simulink model "fibonachi_LFSR"  (R2024a)
settings: Solver=VariableStepAuto  StartTime=0.0  StopTime=1  RelTol=1e-3
values from neighbouring files (symbols this model uses):
  Ts = 1/Fs    (= 7.50007500075e-06)    [new_generation_coeff.m]    (also in simon_test.m; simple_fft_test.m = 1/F; testPSD_c2d.m; testPSD_simulink.m)
libraries: hdlsllib x10, embmathops x7
settings Model: Creator=Simon  LastModifiedBy=Simon

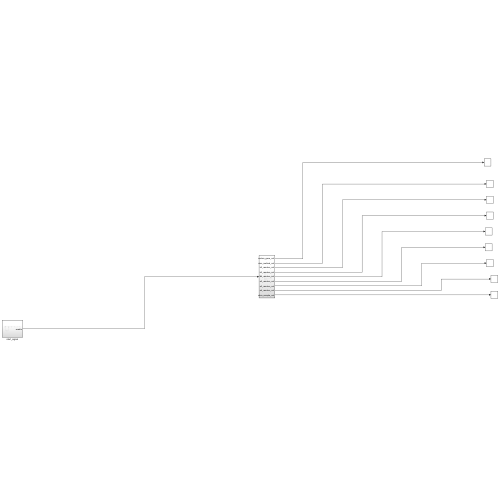
[thumbnail: Simulink's stored preview of the top-level diagram]
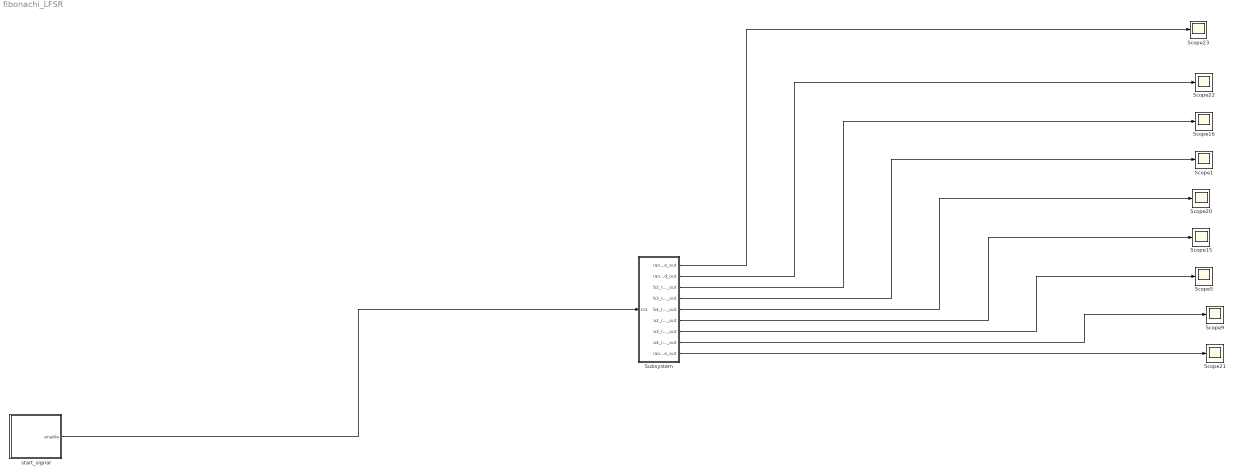
== system fibonachi_LFSR ==
  Scope{1,5,9,15..16,20..23} (9 alike) : Scope
  Subsystem : Subsystem
  start_signal : Subsystem
  wires:
  start_signal/1(enable) -> Subsystem/1(In1)
  Subsystem/1(random_gene_out) -> Scope23/1
  Subsystem/2(random_method_out) -> Scope22/1
  Subsystem/3(b2_random_out) -> Scope16/1
  Subsystem/4(b3_random_out) -> Scope1/1
  Subsystem/5(b4_random_out) -> Scope20/1
  Subsystem/6(a2_random_out) -> Scope15/1
  Subsystem/7(a3_random_out) -> Scope5/1
  Subsystem/8(a4_random_out) -> Scope9/1
  Subsystem/9(random_sample_out) -> Scope21/1

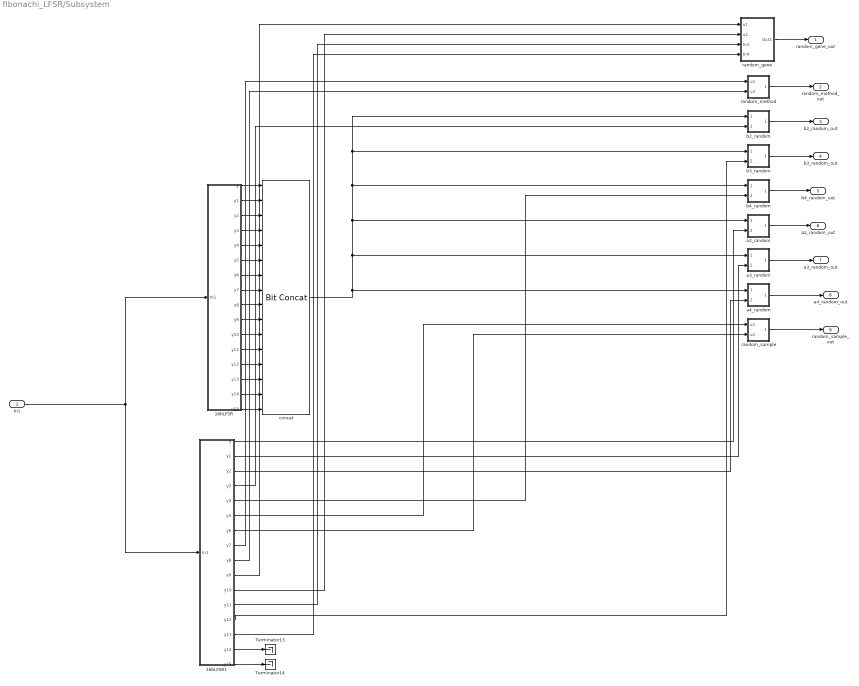
== system fibonachi_LFSR/Subsystem ==
  In1 : Inport
  16bLFSR : Subsystem
  16bLFSR1 : Subsystem
  Terminator13 : Terminator
  Terminator14 : Terminator
  a2_random : Subsystem
  a3_random : Subsystem
  a4_random : Subsystem
  b2_random : Subsystem
  b3_random : Subsystem
  b4_random : Subsystem
  concat : hdlsllib/Logic and Bit Operations/Bit Concat  numInputs=16
  random_gene : Subsystem
  random_method : Subsystem
  random_sample : Subsystem
  random_gene_out : Outport
  random_method_out : Outport  Port=2
  b2_random_out : Outport  Port=3
  b3_random_out : Outport  Port=4
  b4_random_out : Outport  Port=5
  a2_random_out : Outport  Port=6
  a3_random_out : Outport  Port=7
  a4_random_out : Outport  Port=8
  random_sample_out : Outport  Port=9
  wires:
  16bLFSR/11(y10) -> concat/11
  16bLFSR1/10(y9) -> random_gene/1(u1)
  16bLFSR/5(y4) -> concat/5
  16bLFSR/10(y9) -> concat/10
  In1/1 -> 16bLFSR1/1(In1), 16bLFSR/1(In1)
  16bLFSR1/9(y8) -> random_method/2(u2)
  16bLFSR1/12(y11) -> random_gene/3(In3)
  concat/1 -> a3_random/1(In1), a2_random/1(In1), b3_random/1(In1), b2_random/1(In1), b4_random/1(In1), a4_random/1(In1)
  16bLFSR1/13(y12) -> b3_random/2(In2)
  a4_random/1(Out1) -> a4_random_out/1
  16bLFSR/1(y) -> concat/1
  16bLFSR/6(y5) -> concat/6
  16bLFSR1/11(y10) -> random_gene/2(u2)
  random_gene/1(Out1) -> random_gene_out/1
  16bLFSR/14(y13) -> concat/14
  16bLFSR1/14(y13) -> random_gene/4(In4)
  16bLFSR/12(y11) -> concat/12
  a3_random/1(Out1) -> a3_random_out/1
  16bLFSR1/3(y2) -> a4_random/2(In2)
  16bLFSR/4(y3) -> concat/4
  16bLFSR/13(y12) -> concat/13
  16bLFSR/16(y15) -> concat/16
  random_method/1(Out1) -> random_method_out/1
  16bLFSR1/6(y5) -> random_sample/1(u1)
  16bLFSR/2(y1) -> concat/2
  16bLFSR/3(y2) -> concat/3
  16bLFSR1/8(y7) -> random_method/1(u1)
  b2_random/1(Out1) -> b2_random_out/1
  16bLFSR/15(y14) -> concat/15
  16bLFSR1/2(y1) -> a3_random/2(In2)
  16bLFSR1/7(y6) -> random_sample/2(u2)
  16bLFSR1/1(y) -> a2_random/2(In2)
  16bLFSR1/5(y4) -> b4_random/2(In2)
  16bLFSR1/15(y14) -> Terminator13/1
  16bLFSR/8(y7) -> concat/8
  a2_random/1(Out1) -> a2_random_out/1
  random_sample/1(Out1) -> random_sample_out/1
  16bLFSR/9(y8) -> concat/9
  b4_random/1(Out1) -> b4_random_out/1
  16bLFSR/7(y6) -> concat/7
  16bLFSR1/16(y15) -> Terminator14/1
  16bLFSR1/4(y3) -> b2_random/2(In2)
  b3_random/1(Out1) -> b3_random_out/1

== system fibonachi_LFSR/start_signal ==
  Data Type Conversion29 : DataTypeConversion  OutDataTypeStr=boolean  SaturateOnIntegerOverflow=off  RndMeth=Floor
  Delay2 : Delay  DelayLength=1  InitialCondition=0  SampleTime=Ts
  Gain : Gain
  Step1 : Step  Time=Ts*1  SampleTime=Ts
  XOR1 : Logic  Operator=XOR  IconShape=distinctive  AllPortsSameDT=off  OutDataTypeStr=boolean
  enable : Outport
  wires:
  XOR1/1 -> Gain/1
  Step1/1 -> Delay2/1, XOR1/1
  Delay2/1 -> XOR1/2
  Gain/1 -> Data Type Conversion29/1
  Data Type Conversion29/1 -> enable/1

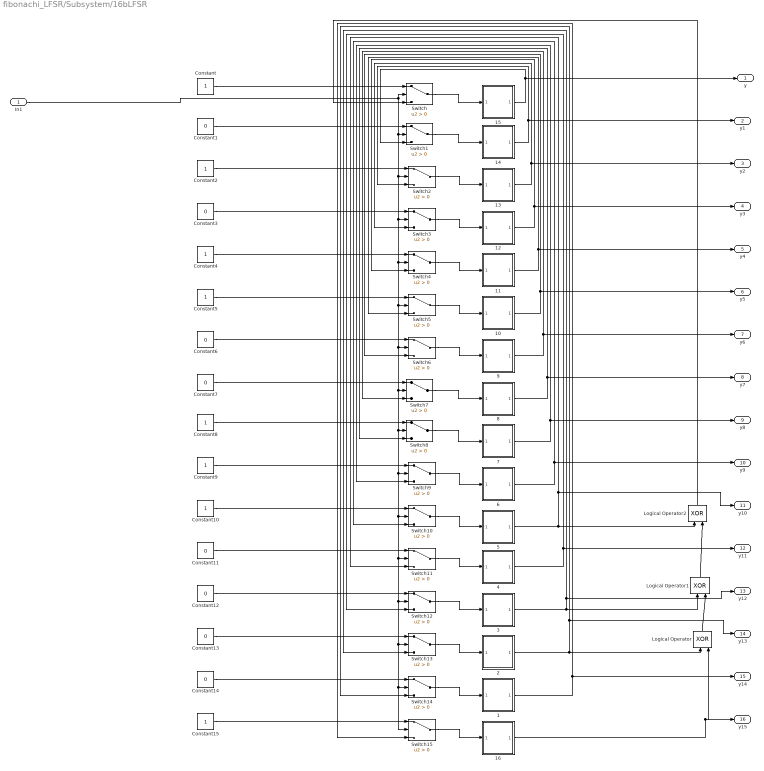
== system fibonachi_LFSR/Subsystem/16bLFSR ==
  In1 : Inport
  1 : Subsystem
  10 : Subsystem
  11 : Subsystem
  12 : Subsystem
  13 : Subsystem
  14 : Subsystem
  15 : Subsystem
  16 : Subsystem
  2 : Subsystem
  3 : Subsystem
  4 : Subsystem
  5 : Subsystem
  6 : Subsystem
  7 : Subsystem
  8 : Subsystem
  9 : Subsystem
  Constant{,2,4..5,8..10,15} (8 alike) : Constant  OutDataTypeStr=boolean  SampleTime=Ts
  Constant{1,3,6..7,11..14} (8 alike) : Constant  Value=0  OutDataTypeStr=boolean  SampleTime=Ts
  Logical Operator : Logic  Operator=XOR  IconShape=distinctive  AllPortsSameDT=off  OutDataTypeStr=boolean
  Logical Operator1 : Logic  Operator=XOR  IconShape=distinctive  AllPortsSameDT=off  OutDataTypeStr=boolean
  Logical Operator2 : Logic  Operator=XOR  IconShape=distinctive  AllPortsSameDT=off  OutDataTypeStr=boolean
  Switch{,1..15} (16 alike) : Switch  Criteria=u2 > Threshold  SaturateOnIntegerOverflow=off  InputSameDT=off
  y : Outport
  y1 : Outport  Port=2
  y2 : Outport  Port=3
  y3 : Outport  Port=4
  y4 : Outport  Port=5
  y5 : Outport  Port=6
  y6 : Outport  Port=7
  y7 : Outport  Port=8
  y8 : Outport  Port=9
  y9 : Outport  Port=10
  y10 : Outport  Port=11
  y11 : Outport  Port=12
  y12 : Outport  Port=13
  y13 : Outport  Port=14
  y14 : Outport  Port=15
  y15 : Outport  Port=16
  wires:
  5/1(reg_out) -> Logical Operator2/1, y10/1, Switch11/3
  6/1(reg_out) -> y9/1, Switch10/3
  2/1(reg_out) -> Logical Operator/1, y13/1, Switch14/3
  11/1(reg_out) -> y4/1, Switch5/3
  Logical Operator2/1 -> Switch/3
  Constant13/1 -> Switch13/1
  Switch13/1 -> 2/1(reg_in)
  3/1(reg_out) -> Logical Operator1/1, y12/1, Switch13/3
  4/1(reg_out) -> y11/1, Switch12/3
  Constant/1 -> Switch/1
  Constant4/1 -> Switch4/1
  Constant2/1 -> Switch2/1
  In1/1 -> Switch/2, Switch15/2, Switch14/2, Switch13/2, Switch12/2, Switch11/2, Switch10/2, Switch9/2, Switch8/2, Switch7/2, Switch6/2, Switch5/2, Switch4/2, Switch3/2, Switch2/2, Switch1/2
  Switch12/1 -> 3/1(reg_in)
  15/1(reg_out) -> y/1, Switch1/3
  Switch1/1 -> 14/1(reg_in)
  Constant8/1 -> Switch8/1
  Constant6/1 -> Switch6/1
  Constant5/1 -> Switch5/1
  Constant14/1 -> Switch14/1
  Constant11/1 -> Switch11/1
  Switch5/1 -> 10/1(reg_in)
  Constant9/1 -> Switch9/1
  Logical Operator/1 -> Logical Operator1/2
  Switch2/1 -> 13/1(reg_in)
  7/1(reg_out) -> y8/1, Switch9/3
  Logical Operator1/1 -> Logical Operator2/2
  Switch11/1 -> 4/1(reg_in)
  Constant7/1 -> Switch7/1
  Switch6/1 -> 9/1(reg_in)
  Switch/1 -> 15/1(reg_in)
  Constant12/1 -> Switch12/1
  Switch4/1 -> 11/1(reg_in)
  Constant15/1 -> Switch15/1
  16/1(reg_out) -> y15/1, Logical Operator/2
  13/1(reg_out) -> y2/1, Switch3/3
  Switch9/1 -> 6/1(reg_in)
  Switch7/1 -> 8/1(reg_in)
  Constant10/1 -> Switch10/1
  Switch14/1 -> 1/1(reg_in)
  Switch3/1 -> 12/1(reg_in)
  Switch15/1 -> 16/1(reg_in)
  9/1(reg_out) -> y6/1, Switch7/3
  Constant3/1 -> Switch3/1
  Constant1/1 -> Switch1/1
  14/1(reg_out) -> y1/1, Switch2/3
  Switch10/1 -> 5/1(reg_in)
  10/1(reg_out) -> y5/1, Switch6/3
  Switch8/1 -> 7/1(reg_in)
  12/1(reg_out) -> y3/1, Switch4/3
  8/1(reg_out) -> y7/1, Switch8/3
  1/1(reg_out) -> y14/1, Switch15/3

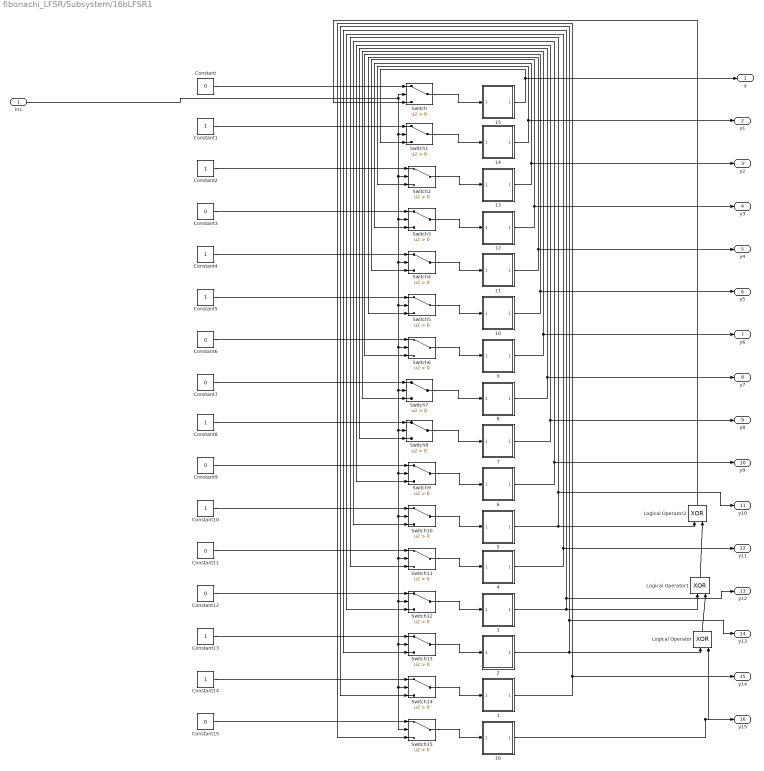
== system fibonachi_LFSR/Subsystem/16bLFSR1 ==
  In1 : Inport
  1 : Subsystem
  10 : Subsystem
  11 : Subsystem
  12 : Subsystem
  13 : Subsystem
  14 : Subsystem
  15 : Subsystem
  16 : Subsystem
  2 : Subsystem
  3 : Subsystem
  4 : Subsystem
  5 : Subsystem
  6 : Subsystem
  7 : Subsystem
  8 : Subsystem
  9 : Subsystem
  Constant{,3,6..7,9,11..12,15} (8 alike) : Constant  Value=0  OutDataTypeStr=boolean  SampleTime=Ts
  Constant{1..2,4..5,8,10,13..14} (8 alike) : Constant  OutDataTypeStr=boolean  SampleTime=Ts
  Logical Operator : Logic  Operator=XOR  IconShape=distinctive  AllPortsSameDT=off  OutDataTypeStr=boolean
  Logical Operator1 : Logic  Operator=XOR  IconShape=distinctive  AllPortsSameDT=off  OutDataTypeStr=boolean
  Logical Operator2 : Logic  Operator=XOR  IconShape=distinctive  AllPortsSameDT=off  OutDataTypeStr=boolean
  Switch{,1..15} (16 alike) : Switch  Criteria=u2 > Threshold  SaturateOnIntegerOverflow=off  InputSameDT=off
  y : Outport
  y1 : Outport  Port=2
  y2 : Outport  Port=3
  y3 : Outport  Port=4
  y4 : Outport  Port=5
  y5 : Outport  Port=6
  y6 : Outport  Port=7
  y7 : Outport  Port=8
  y8 : Outport  Port=9
  y9 : Outport  Port=10
  y10 : Outport  Port=11
  y11 : Outport  Port=12
  y12 : Outport  Port=13
  y13 : Outport  Port=14
  y14 : Outport  Port=15
  y15 : Outport  Port=16
  wires:
  1/1(reg_out) -> Switch15/3, y14/1
  8/1(reg_out) -> Switch8/3, y7/1
  12/1(reg_out) -> Switch4/3, y3/1
  Switch8/1 -> 7/1(reg_in)
  10/1(reg_out) -> Switch6/3, y5/1
  Switch10/1 -> 5/1(reg_in)
  14/1(reg_out) -> Switch2/3, y1/1
  Constant1/1 -> Switch1/1
  Constant3/1 -> Switch3/1
  9/1(reg_out) -> Switch7/3, y6/1
  Switch15/1 -> 16/1(reg_in)
  Switch3/1 -> 12/1(reg_in)
  Switch14/1 -> 1/1(reg_in)
  Constant10/1 -> Switch10/1
  Switch7/1 -> 8/1(reg_in)
  Switch9/1 -> 6/1(reg_in)
  13/1(reg_out) -> Switch3/3, y2/1
  16/1(reg_out) -> Logical Operator/2, y15/1
  Constant15/1 -> Switch15/1
  Switch4/1 -> 11/1(reg_in)
  Constant12/1 -> Switch12/1
  Switch/1 -> 15/1(reg_in)
  Switch6/1 -> 9/1(reg_in)
  Constant7/1 -> Switch7/1
  Switch11/1 -> 4/1(reg_in)
  Logical Operator1/1 -> Logical Operator2/2
  7/1(reg_out) -> Switch9/3, y8/1
  Switch2/1 -> 13/1(reg_in)
  Logical Operator/1 -> Logical Operator1/2
  Constant9/1 -> Switch9/1
  Switch5/1 -> 10/1(reg_in)
  Constant11/1 -> Switch11/1
  Constant14/1 -> Switch14/1
  Constant5/1 -> Switch5/1
  Constant6/1 -> Switch6/1
  Constant8/1 -> Switch8/1
  Switch1/1 -> 14/1(reg_in)
  15/1(reg_out) -> Switch1/3, y/1
  Switch12/1 -> 3/1(reg_in)
  In1/1 -> Switch1/2, Switch2/2, Switch3/2, Switch4/2, Switch5/2, Switch6/2, Switch7/2, Switch8/2, Switch9/2, Switch10/2, Switch11/2, Switch12/2, Switch13/2, Switch14/2, Switch15/2, Switch/2
  Constant2/1 -> Switch2/1
  Constant4/1 -> Switch4/1
  Constant/1 -> Switch/1
  4/1(reg_out) -> Switch12/3, y11/1
  3/1(reg_out) -> Switch13/3, y12/1, Logical Operator1/1
  Switch13/1 -> 2/1(reg_in)
  Constant13/1 -> Switch13/1
  Logical Operator2/1 -> Switch/3
  11/1(reg_out) -> Switch5/3, y4/1
  2/1(reg_out) -> Switch14/3, y13/1, Logical Operator/1
  6/1(reg_out) -> Switch10/3, y9/1
  5/1(reg_out) -> Switch11/3, y10/1, Logical Operator2/1

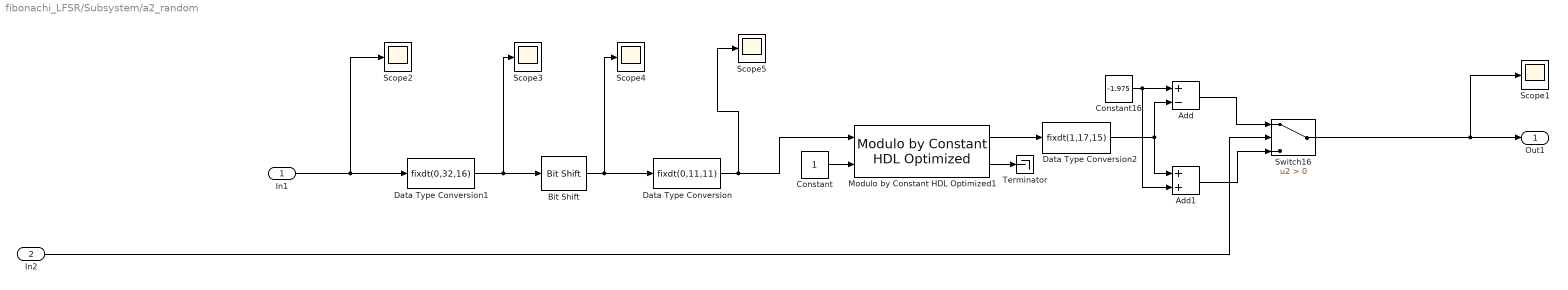
== system fibonachi_LFSR/Subsystem/a2_random ==
  In1 : Inport
  In2 : Inport  Port=2
  Add : Sum  Inputs=+-  OutDataTypeStr=Inherit: Same as first input
  Add1 : Sum  OutDataTypeStr=Inherit: Same as first input
  Bit Shift : hdlsllib/Logic and Bit Operations/Bit Shift  mode=Shift Right Logical  N=16+5
  Constant : Constant  OutDataTypeStr=boolean  SampleTime=Ts
  Constant16 : Constant  Value=-1.975  OutDataTypeStr=fixdt(1,17,15)  SampleTime=Ts
  Data Type Conversion : DataTypeConversion  OutDataTypeStr=fixdt(0,11,11)  SaturateOnIntegerOverflow=off  RndMeth=Floor
  Data Type Conversion1 : DataTypeConversion  OutDataTypeStr=fixdt(0,32,16)  SaturateOnIntegerOverflow=off  RndMeth=Floor
  Data Type Conversion2 : DataTypeConversion  OutDataTypeStr=fixdt(1,17,15)  SaturateOnIntegerOverflow=off  RndMeth=Floor
  Modulo by Constant HDL Optimized1 : embmathops/Modulo by Constant HDL Optimized  Denominator=0.025  SimulateUsing=Code generation
      settings: LibrarySourceBlock=|
      | embeddedMatrixLib/Math Operations/Modulo by Constant
      | HDL Optimized
  Scope{1..5} (5 alike) : Scope
  Switch16 : Switch  Criteria=u2 > Threshold  SaturateOnIntegerOverflow=off  InputSameDT=off
  Terminator : Terminator
  Out1 : Outport
  wires:
  Data Type Conversion2/1 -> Add/2, Add1/1
  Bit Shift/1 -> Scope4/1, Data Type Conversion/1
  Add1/1 -> Switch16/3
  Add/1 -> Switch16/1
  Data Type Conversion1/1 -> Scope3/1, Bit Shift/1
  Constant16/1 -> Add1/2, Add/1
  Switch16/1 -> Scope1/1, Out1/1
  Data Type Conversion/1 -> Modulo by Constant HDL Optimized1/1, Scope5/1
  In2/1 -> Switch16/2
  In1/1 -> Scope2/1, Data Type Conversion1/1
  Constant/1 -> Modulo by Constant HDL Optimized1/2
  Modulo by Constant HDL Optimized1/2 -> Terminator/1
  Modulo by Constant HDL Optimized1/1 -> Data Type Conversion2/1

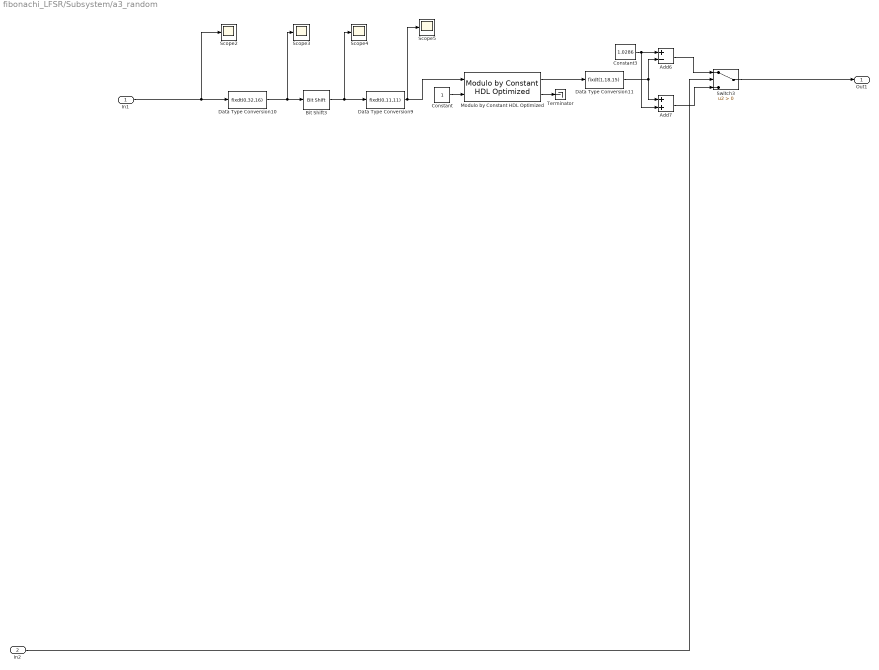
== system fibonachi_LFSR/Subsystem/a3_random ==
  In1 : Inport
  In2 : Inport  Port=2
  Add6 : Sum  Inputs=+-  OutDataTypeStr=Inherit: Same as first input
  Add7 : Sum  OutDataTypeStr=Inherit: Same as first input
  Bit Shift3 : hdlsllib/Logic and Bit Operations/Bit Shift  mode=Shift Right Logical  N=16+6
  Constant : Constant  OutDataTypeStr=boolean  SampleTime=Ts
  Constant3 : Constant  Value=1.0286  OutDataTypeStr=fixdt(1,18,15)  SampleTime=Ts
  Data Type Conversion10 : DataTypeConversion  OutDataTypeStr=fixdt(0,32,16)  SaturateOnIntegerOverflow=off  RndMeth=Floor
  Data Type Conversion11 : DataTypeConversion  OutDataTypeStr=fixdt(1,18,15)  SaturateOnIntegerOverflow=off  RndMeth=Floor
  Data Type Conversion9 : DataTypeConversion  OutDataTypeStr=fixdt(0,11,11)  SaturateOnIntegerOverflow=off  RndMeth=Floor
  Modulo by Constant HDL Optimized : embmathops/Modulo by Constant HDL Optimized  Denominator=0.0106  SimulateUsing=Code generation
      settings: LibrarySourceBlock=|
      | embeddedMatrixLib/Math Operations/Modulo by Constant
      | HDL Optimized
  Scope{2..5} (4 alike) : Scope
  Switch3 : Switch  Criteria=u2 > Threshold  SaturateOnIntegerOverflow=off  InputSameDT=off
  Terminator : Terminator
  Out1 : Outport
  wires:
  Constant3/1 -> Add6/1, Add7/2
  Modulo by Constant HDL Optimized/1 -> Data Type Conversion11/1
  Add6/1 -> Switch3/1
  Data Type Conversion11/1 -> Add7/1, Add6/2
  Add7/1 -> Switch3/3
  In2/1 -> Switch3/2
  Switch3/1 -> Out1/1
  In1/1 -> Scope2/1, Data Type Conversion10/1
  Bit Shift3/1 -> Scope4/1, Data Type Conversion9/1
  Data Type Conversion9/1 -> Modulo by Constant HDL Optimized/1, Scope5/1
  Data Type Conversion10/1 -> Scope3/1, Bit Shift3/1
  Constant/1 -> Modulo by Constant HDL Optimized/2
  Modulo by Constant HDL Optimized/2 -> Terminator/1

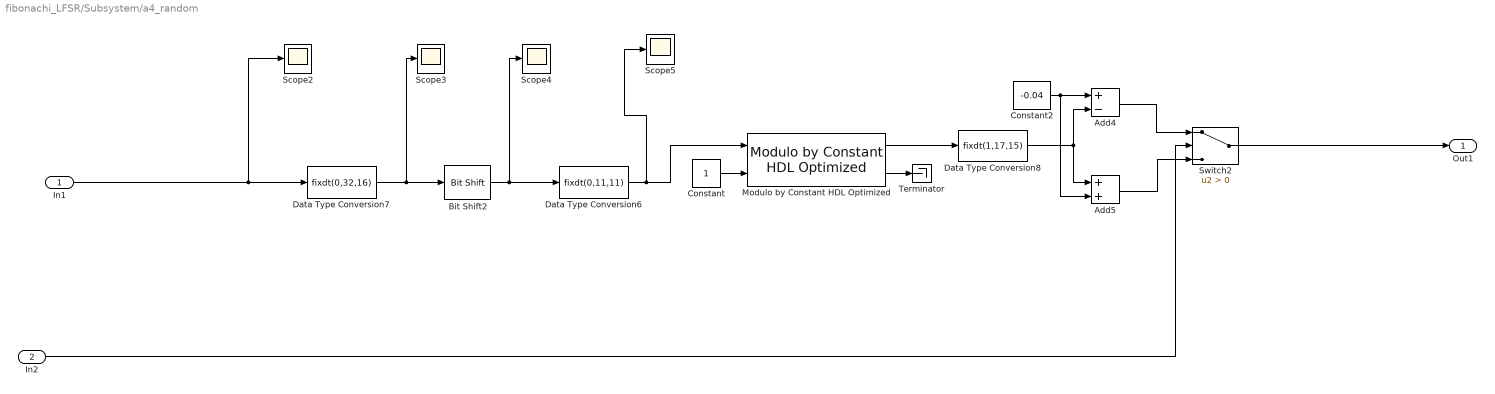
== system fibonachi_LFSR/Subsystem/a4_random ==
  In1 : Inport
  In2 : Inport  Port=2
  Add4 : Sum  Inputs=+-  OutDataTypeStr=Inherit: Same as first input
  Add5 : Sum  OutDataTypeStr=Inherit: Same as first input
  Bit Shift2 : hdlsllib/Logic and Bit Operations/Bit Shift  mode=Shift Right Logical  N=16+6
  Constant : Constant  OutDataTypeStr=boolean  SampleTime=Ts
  Constant2 : Constant  Value=-0.04  OutDataTypeStr=fixdt(1,17,15)  SampleTime=Ts
  Data Type Conversion6 : DataTypeConversion  OutDataTypeStr=fixdt(0,11,11)  SaturateOnIntegerOverflow=off  RndMeth=Floor
  Data Type Conversion7 : DataTypeConversion  OutDataTypeStr=fixdt(0,32,16)  SaturateOnIntegerOverflow=off  RndMeth=Floor
  Data Type Conversion8 : DataTypeConversion  OutDataTypeStr=fixdt(1,17,15)  SaturateOnIntegerOverflow=off  RndMeth=Floor
  Modulo by Constant HDL Optimized : embmathops/Modulo by Constant HDL Optimized  Denominator=0.008  SimulateUsing=Code generation
      settings: LibrarySourceBlock=|
      | embeddedMatrixLib/Math Operations/Modulo by Constant
      | HDL Optimized
  Scope{2..5} (4 alike) : Scope
  Switch2 : Switch  Criteria=u2 > Threshold  SaturateOnIntegerOverflow=off  InputSameDT=off
  Terminator : Terminator
  Out1 : Outport
  wires:
  Data Type Conversion8/1 -> Add4/2, Add5/1
  Modulo by Constant HDL Optimized/1 -> Data Type Conversion8/1
  Constant2/1 -> Add5/2, Add4/1
  In2/1 -> Switch2/2
  Add4/1 -> Switch2/1
  Add5/1 -> Switch2/3
  Switch2/1 -> Out1/1
  In1/1 -> Scope2/1, Data Type Conversion7/1
  Bit Shift2/1 -> Scope4/1, Data Type Conversion6/1
  Data Type Conversion6/1 -> Modulo by Constant HDL Optimized/1, Scope5/1
  Data Type Conversion7/1 -> Scope3/1, Bit Shift2/1
  Constant/1 -> Modulo by Constant HDL Optimized/2
  Modulo by Constant HDL Optimized/2 -> Terminator/1

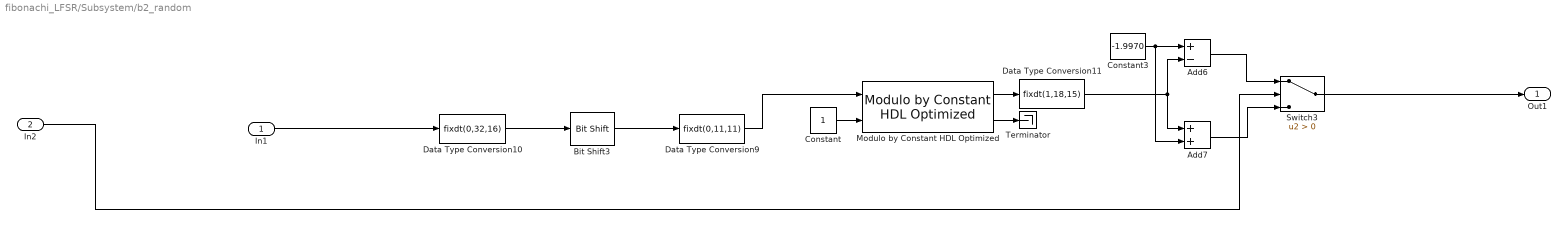
== system fibonachi_LFSR/Subsystem/b2_random ==
  In1 : Inport
  In2 : Inport  Port=2
  Add6 : Sum  Inputs=+-  OutDataTypeStr=Inherit: Same as first input
  Add7 : Sum  OutDataTypeStr=Inherit: Same as first input
  Bit Shift3 : hdlsllib/Logic and Bit Operations/Bit Shift  mode=Shift Right Logical  N=16+6
  Constant : Constant  OutDataTypeStr=boolean  SampleTime=Ts
  Constant3 : Constant  Value=-1.9970  OutDataTypeStr=fixdt(1,18,15)  SampleTime=Ts
  Data Type Conversion10 : DataTypeConversion  OutDataTypeStr=fixdt(0,32,16)  SaturateOnIntegerOverflow=off  RndMeth=Floor
  Data Type Conversion11 : DataTypeConversion  OutDataTypeStr=fixdt(1,18,15)  SaturateOnIntegerOverflow=off  RndMeth=Floor
  Data Type Conversion9 : DataTypeConversion  OutDataTypeStr=fixdt(0,11,11)  RndMeth=Floor
  Modulo by Constant HDL Optimized : embmathops/Modulo by Constant HDL Optimized  Denominator=0.0130  SimulateUsing=Code generation
      settings: LibrarySourceBlock=|
      | embeddedMatrixLib/Math Operations/Modulo by Constant
      | HDL Optimized
  Switch3 : Switch  Criteria=u2 > Threshold  SaturateOnIntegerOverflow=off  InputSameDT=off
  Terminator : Terminator
  Out1 : Outport
  wires:
  Constant3/1 -> Add6/1, Add7/2
  Modulo by Constant HDL Optimized/1 -> Data Type Conversion11/1
  Add6/1 -> Switch3/1
  Data Type Conversion11/1 -> Add7/1, Add6/2
  Add7/1 -> Switch3/3
  In2/1 -> Switch3/2
  Switch3/1 -> Out1/1
  In1/1 -> Data Type Conversion10/1
  Bit Shift3/1 -> Data Type Conversion9/1
  Data Type Conversion9/1 -> Modulo by Constant HDL Optimized/1
  Data Type Conversion10/1 -> Bit Shift3/1
  Constant/1 -> Modulo by Constant HDL Optimized/2
  Modulo by Constant HDL Optimized/2 -> Terminator/1

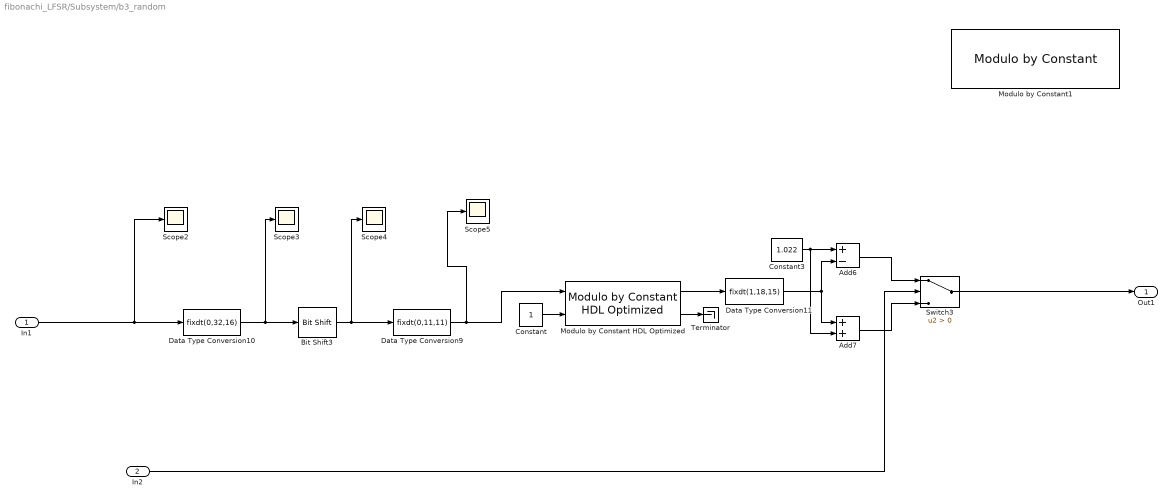
== system fibonachi_LFSR/Subsystem/b3_random ==
  In1 : Inport
  In2 : Inport  Port=2
  Add6 : Sum  Inputs=+-  OutDataTypeStr=Inherit: Same as first input
  Add7 : Sum  OutDataTypeStr=Inherit: Same as first input
  Bit Shift3 : hdlsllib/Logic and Bit Operations/Bit Shift  mode=Shift Right Logical  N=16+6
  Constant : Constant  OutDataTypeStr=boolean  SampleTime=Ts
  Constant3 : Constant  Value=1.022  OutDataTypeStr=fixdt(1,18,15)  SampleTime=Ts
  Data Type Conversion10 : DataTypeConversion  OutDataTypeStr=fixdt(0,32,16)  SaturateOnIntegerOverflow=off  RndMeth=Floor
  Data Type Conversion11 : DataTypeConversion  OutDataTypeStr=fixdt(1,18,15)  SaturateOnIntegerOverflow=off  RndMeth=Floor
  Data Type Conversion9 : DataTypeConversion  OutDataTypeStr=fixdt(0,11,11)  RndMeth=Floor
  Modulo by Constant HDL Optimized : embmathops/Modulo by Constant HDL Optimized  Denominator=0.01  SimulateUsing=Code generation
      settings: LibrarySourceBlock=|
      | embeddedMatrixLib/Math Operations/Modulo by Constant
      | HDL Optimized
  Modulo by Constant1 : embmathops/Modulo by Constant  Denominator=0.01  SimulateUsing=Code generation
      settings: LibrarySourceBlock=embeddedMathLib/Modulo by Constant
  Scope{2..5} (4 alike) : Scope
  Switch3 : Switch  Criteria=u2 > Threshold  SaturateOnIntegerOverflow=off  InputSameDT=off
  Terminator : Terminator
  Out1 : Outport
  wires:
  Switch3/1 -> Out1/1
  In2/1 -> Switch3/2
  Add7/1 -> Switch3/3
  Data Type Conversion11/1 -> Add6/2, Add7/1
  Add6/1 -> Switch3/1
  Modulo by Constant HDL Optimized/1 -> Data Type Conversion11/1
  Constant3/1 -> Add7/2, Add6/1
  In1/1 -> Scope2/1, Data Type Conversion10/1
  Bit Shift3/1 -> Scope4/1, Data Type Conversion9/1
  Data Type Conversion9/1 -> Modulo by Constant HDL Optimized/1, Scope5/1
  Data Type Conversion10/1 -> Scope3/1, Bit Shift3/1
  Constant/1 -> Modulo by Constant HDL Optimized/2
  Modulo by Constant HDL Optimized/2 -> Terminator/1

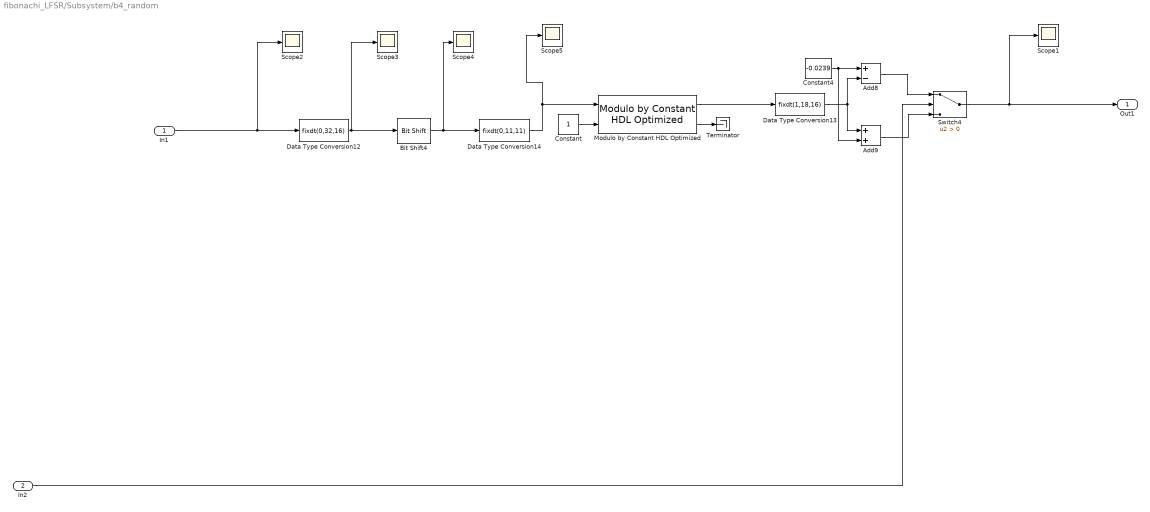
== system fibonachi_LFSR/Subsystem/b4_random ==
  In1 : Inport
  In2 : Inport  Port=2
  Add8 : Sum  Inputs=+-  OutDataTypeStr=Inherit: Same as first input
  Add9 : Sum  OutDataTypeStr=Inherit: Same as first input
  Bit Shift4 : hdlsllib/Logic and Bit Operations/Bit Shift  mode=Shift Right Logical  N=16+12
  Constant : Constant  OutDataTypeStr=boolean  SampleTime=Ts
  Constant4 : Constant  Value=-0.0239  OutDataTypeStr=fixdt(1,18,15)  SampleTime=Ts
  Data Type Conversion12 : DataTypeConversion  OutDataTypeStr=fixdt(0,32,16)  SaturateOnIntegerOverflow=off  RndMeth=Floor
  Data Type Conversion13 : DataTypeConversion  OutDataTypeStr=fixdt(1,18,16)  SaturateOnIntegerOverflow=off  RndMeth=Floor
  Data Type Conversion14 : DataTypeConversion  OutDataTypeStr=fixdt(0,11,11)  SaturateOnIntegerOverflow=off  RndMeth=Floor
  Modulo by Constant HDL Optimized : embmathops/Modulo by Constant HDL Optimized  Denominator=2.5e-4  SimulateUsing=Code generation
      settings: LibrarySourceBlock=|
      | embeddedMatrixLib/Math Operations/Modulo by Constant
      | HDL Optimized
  Scope{1..5} (5 alike) : Scope
  Switch4 : Switch  Criteria=u2 > Threshold  SaturateOnIntegerOverflow=off  InputSameDT=off
  Terminator : Terminator
  Out1 : Outport
  wires:
  Data Type Conversion13/1 -> Add8/2, Add9/1
  Constant4/1 -> Add9/2, Add8/1
  Modulo by Constant HDL Optimized/1 -> Data Type Conversion13/1
  In2/1 -> Switch4/2
  Add9/1 -> Switch4/3
  Add8/1 -> Switch4/1
  Switch4/1 -> Scope1/1, Out1/1
  In1/1 -> Scope2/1, Data Type Conversion12/1
  Bit Shift4/1 -> Scope4/1, Data Type Conversion14/1
  Data Type Conversion14/1 -> Modulo by Constant HDL Optimized/1, Scope5/1
  Data Type Conversion12/1 -> Scope3/1, Bit Shift4/1
  Constant/1 -> Modulo by Constant HDL Optimized/2
  Modulo by Constant HDL Optimized/2 -> Terminator/1

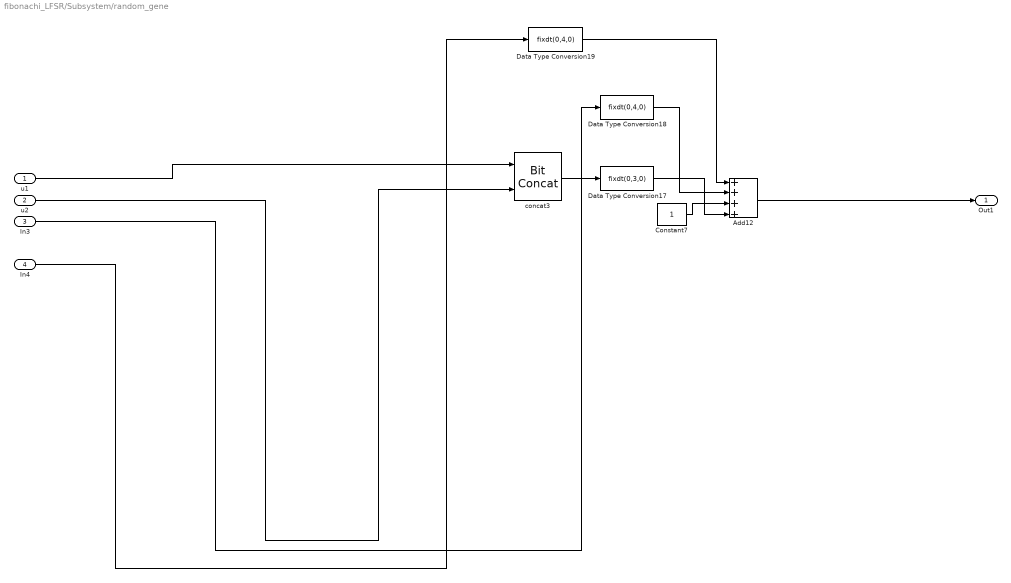
== system fibonachi_LFSR/Subsystem/random_gene ==
  u1 : Inport
  u2 : Inport  Port=2
  In3 : Inport  Port=3
  In4 : Inport  Port=4
  Add12 : Sum  Inputs=++++  OutDataTypeStr=Inherit: Same as first input
  Constant7 : Constant  OutDataTypeStr=fixdt(0,3,0)  SampleTime=Ts
  Data Type Conversion17 : DataTypeConversion  OutDataTypeStr=fixdt(0,3,0)  SaturateOnIntegerOverflow=off  RndMeth=Floor
  Data Type Conversion18 : DataTypeConversion  OutDataTypeStr=fixdt(0,4,0)  SaturateOnIntegerOverflow=off  RndMeth=Floor
  Data Type Conversion19 : DataTypeConversion  OutDataTypeStr=fixdt(0,4,0)  SaturateOnIntegerOverflow=off  RndMeth=Floor
  concat3 : hdlsllib/Logic and Bit Operations/Bit Concat  numInputs=2
  Out1 : Outport
  wires:
  In3/1 -> Data Type Conversion18/1
  Data Type Conversion18/1 -> Add12/2
  u1/1 -> concat3/1
  u2/1 -> concat3/2
  Add12/1 -> Out1/1
  Data Type Conversion17/1 -> Add12/4
  concat3/1 -> Data Type Conversion17/1
  Constant7/1 -> Add12/3
  Data Type Conversion19/1 -> Add12/1
  In4/1 -> Data Type Conversion19/1

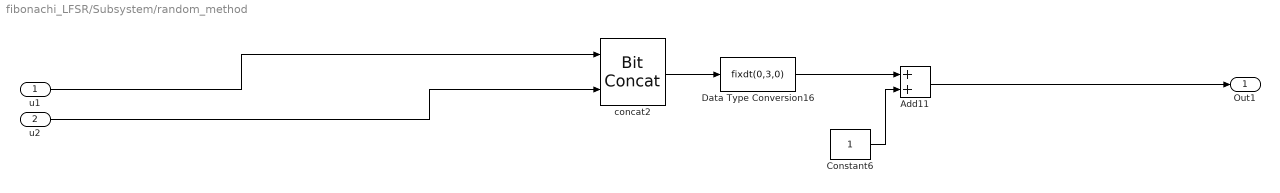
== system fibonachi_LFSR/Subsystem/random_method ==
  u1 : Inport
  u2 : Inport  Port=2
  Add11 : Sum  OutDataTypeStr=Inherit: Same as first input
  Constant6 : Constant  OutDataTypeStr=fixdt(0,3,0)  SampleTime=Ts
  Data Type Conversion16 : DataTypeConversion  OutDataTypeStr=fixdt(0,3,0)  SaturateOnIntegerOverflow=off  RndMeth=Floor
  concat2 : hdlsllib/Logic and Bit Operations/Bit Concat  numInputs=2
  Out1 : Outport
  wires:
  Constant6/1 -> Add11/2
  Add11/1 -> Out1/1
  concat2/1 -> Data Type Conversion16/1
  u1/1 -> concat2/1
  Data Type Conversion16/1 -> Add11/1
  u2/1 -> concat2/2

== system fibonachi_LFSR/Subsystem/random_sample ==
  u1 : Inport
  u2 : Inport  Port=2
  Add10 : Sum  OutDataTypeStr=Inherit: Same as first input
  Constant5 : Constant  OutDataTypeStr=fixdt(0,4,0)  SampleTime=Ts
  Data Type Conversion15 : DataTypeConversion  OutDataTypeStr=fixdt(0,4,0)  SaturateOnIntegerOverflow=off  RndMeth=Floor
  concat1 : hdlsllib/Logic and Bit Operations/Bit Concat  numInputs=2
  Out1 : Outport
  wires:
  Add10/1 -> Out1/1
  Constant5/1 -> Add10/2
  Data Type Conversion15/1 -> Add10/1
  concat1/1 -> Data Type Conversion15/1
  u2/1 -> concat1/2
  u1/1 -> concat1/1

== system fibonachi_LFSR/Subsystem/16bLFSR/1 ==
  reg_in : Inport
  Delay : Delay  DelayLength=1  InitialCondition=0  SampleTime=Ts
  reg_out : Outport
  wires:
  reg_in/1 -> Delay/1
  Delay/1 -> reg_out/1

== system fibonachi_LFSR/Subsystem/16bLFSR/10 ==
  reg_in : Inport
  Delay : Delay  DelayLength=1  InitialCondition=0  SampleTime=Ts
  reg_out : Outport
  wires:
  Delay/1 -> reg_out/1
  reg_in/1 -> Delay/1

== system fibonachi_LFSR/Subsystem/16bLFSR/11 ==
  reg_in : Inport
  Delay : Delay  DelayLength=1  InitialCondition=0  SampleTime=Ts
  reg_out : Outport
  wires:
  reg_in/1 -> Delay/1
  Delay/1 -> reg_out/1

== system fibonachi_LFSR/Subsystem/16bLFSR/12 ==
  reg_in : Inport
  Delay : Delay  DelayLength=1  InitialCondition=0  SampleTime=Ts
  reg_out : Outport
  wires:
  Delay/1 -> reg_out/1
  reg_in/1 -> Delay/1

== system fibonachi_LFSR/Subsystem/16bLFSR/13 ==
  reg_in : Inport
  Delay : Delay  DelayLength=1  InitialCondition=0  SampleTime=Ts
  reg_out : Outport
  wires:
  reg_in/1 -> Delay/1
  Delay/1 -> reg_out/1

== system fibonachi_LFSR/Subsystem/16bLFSR/14 ==
  reg_in : Inport
  Delay : Delay  DelayLength=1  InitialCondition=0  SampleTime=Ts
  reg_out : Outport
  wires:
  Delay/1 -> reg_out/1
  reg_in/1 -> Delay/1

== system fibonachi_LFSR/Subsystem/16bLFSR/15 ==
  reg_in : Inport
  Delay : Delay  DelayLength=1  InitialCondition=0  SampleTime=Ts
  reg_out : Outport
  wires:
  reg_in/1 -> Delay/1
  Delay/1 -> reg_out/1

== system fibonachi_LFSR/Subsystem/16bLFSR/16 ==
  reg_in : Inport
  Delay : Delay  DelayLength=1  InitialCondition=0  SampleTime=Ts
  reg_out : Outport
  wires:
  Delay/1 -> reg_out/1
  reg_in/1 -> Delay/1

== system fibonachi_LFSR/Subsystem/16bLFSR/2 ==
  reg_in : Inport
  Delay : Delay  DelayLength=1  InitialCondition=0  SampleTime=Ts
  reg_out : Outport
  wires:
  Delay/1 -> reg_out/1
  reg_in/1 -> Delay/1

== system fibonachi_LFSR/Subsystem/16bLFSR/3 ==
  reg_in : Inport
  Delay : Delay  DelayLength=1  InitialCondition=0  SampleTime=Ts
  reg_out : Outport
  wires:
  reg_in/1 -> Delay/1
  Delay/1 -> reg_out/1

== system fibonachi_LFSR/Subsystem/16bLFSR/4 ==
  reg_in : Inport
  Delay : Delay  DelayLength=1  InitialCondition=0  SampleTime=Ts
  reg_out : Outport
  wires:
  Delay/1 -> reg_out/1
  reg_in/1 -> Delay/1

== system fibonachi_LFSR/Subsystem/16bLFSR/5 ==
  reg_in : Inport
  Delay : Delay  DelayLength=1  InitialCondition=0  SampleTime=Ts
  reg_out : Outport
  wires:
  reg_in/1 -> Delay/1
  Delay/1 -> reg_out/1

== system fibonachi_LFSR/Subsystem/16bLFSR/6 ==
  reg_in : Inport
  Delay : Delay  DelayLength=1  InitialCondition=0  SampleTime=Ts
  reg_out : Outport
  wires:
  Delay/1 -> reg_out/1
  reg_in/1 -> Delay/1

== system fibonachi_LFSR/Subsystem/16bLFSR/7 ==
  reg_in : Inport
  Delay : Delay  DelayLength=1  InitialCondition=0  SampleTime=Ts
  reg_out : Outport
  wires:
  reg_in/1 -> Delay/1
  Delay/1 -> reg_out/1

== system fibonachi_LFSR/Subsystem/16bLFSR/8 ==
  reg_in : Inport
  Delay : Delay  DelayLength=1  InitialCondition=0  SampleTime=Ts
  reg_out : Outport
  wires:
  Delay/1 -> reg_out/1
  reg_in/1 -> Delay/1

== system fibonachi_LFSR/Subsystem/16bLFSR/9 ==
  reg_in : Inport
  Delay : Delay  DelayLength=1  InitialCondition=0  SampleTime=Ts
  reg_out : Outport
  wires:
  reg_in/1 -> Delay/1
  Delay/1 -> reg_out/1

== system fibonachi_LFSR/Subsystem/16bLFSR1/1 ==
  reg_in : Inport
  Delay : Delay  DelayLength=1  InitialCondition=0  SampleTime=Ts
  reg_out : Outport
  wires:
  Delay/1 -> reg_out/1
  reg_in/1 -> Delay/1

== system fibonachi_LFSR/Subsystem/16bLFSR1/10 ==
  reg_in : Inport
  Delay : Delay  DelayLength=1  InitialCondition=0  SampleTime=Ts
  reg_out : Outport
  wires:
  reg_in/1 -> Delay/1
  Delay/1 -> reg_out/1

== system fibonachi_LFSR/Subsystem/16bLFSR1/11 ==
  reg_in : Inport
  Delay : Delay  DelayLength=1  InitialCondition=0  SampleTime=Ts
  reg_out : Outport
  wires:
  Delay/1 -> reg_out/1
  reg_in/1 -> Delay/1

== system fibonachi_LFSR/Subsystem/16bLFSR1/12 ==
  reg_in : Inport
  Delay : Delay  DelayLength=1  InitialCondition=0  SampleTime=Ts
  reg_out : Outport
  wires:
  reg_in/1 -> Delay/1
  Delay/1 -> reg_out/1

== system fibonachi_LFSR/Subsystem/16bLFSR1/13 ==
  reg_in : Inport
  Delay : Delay  DelayLength=1  InitialCondition=0  SampleTime=Ts
  reg_out : Outport
  wires:
  Delay/1 -> reg_out/1
  reg_in/1 -> Delay/1

== system fibonachi_LFSR/Subsystem/16bLFSR1/14 ==
  reg_in : Inport
  Delay : Delay  DelayLength=1  InitialCondition=0  SampleTime=Ts
  reg_out : Outport
  wires:
  reg_in/1 -> Delay/1
  Delay/1 -> reg_out/1

== system fibonachi_LFSR/Subsystem/16bLFSR1/15 ==
  reg_in : Inport
  Delay : Delay  DelayLength=1  InitialCondition=0  SampleTime=Ts
  reg_out : Outport
  wires:
  Delay/1 -> reg_out/1
  reg_in/1 -> Delay/1

== system fibonachi_LFSR/Subsystem/16bLFSR1/16 ==
  reg_in : Inport
  Delay : Delay  DelayLength=1  InitialCondition=0  SampleTime=Ts
  reg_out : Outport
  wires:
  reg_in/1 -> Delay/1
  Delay/1 -> reg_out/1

== system fibonachi_LFSR/Subsystem/16bLFSR1/2 ==
  reg_in : Inport
  Delay : Delay  DelayLength=1  InitialCondition=0  SampleTime=Ts
  reg_out : Outport
  wires:
  reg_in/1 -> Delay/1
  Delay/1 -> reg_out/1

== system fibonachi_LFSR/Subsystem/16bLFSR1/3 ==
  reg_in : Inport
  Delay : Delay  DelayLength=1  InitialCondition=0  SampleTime=Ts
  reg_out : Outport
  wires:
  Delay/1 -> reg_out/1
  reg_in/1 -> Delay/1

== system fibonachi_LFSR/Subsystem/16bLFSR1/4 ==
  reg_in : Inport
  Delay : Delay  DelayLength=1  InitialCondition=0  SampleTime=Ts
  reg_out : Outport
  wires:
  reg_in/1 -> Delay/1
  Delay/1 -> reg_out/1

== system fibonachi_LFSR/Subsystem/16bLFSR1/5 ==
  reg_in : Inport
  Delay : Delay  DelayLength=1  InitialCondition=0  SampleTime=Ts
  reg_out : Outport
  wires:
  Delay/1 -> reg_out/1
  reg_in/1 -> Delay/1

== system fibonachi_LFSR/Subsystem/16bLFSR1/6 ==
  reg_in : Inport
  Delay : Delay  DelayLength=1  InitialCondition=0  SampleTime=Ts
  reg_out : Outport
  wires:
  reg_in/1 -> Delay/1
  Delay/1 -> reg_out/1

== system fibonachi_LFSR/Subsystem/16bLFSR1/7 ==
  reg_in : Inport
  Delay : Delay  DelayLength=1  InitialCondition=0  SampleTime=Ts
  reg_out : Outport
  wires:
  Delay/1 -> reg_out/1
  reg_in/1 -> Delay/1

== system fibonachi_LFSR/Subsystem/16bLFSR1/8 ==
  reg_in : Inport
  Delay : Delay  DelayLength=1  InitialCondition=0  SampleTime=Ts
  reg_out : Outport
  wires:
  reg_in/1 -> Delay/1
  Delay/1 -> reg_out/1

== system fibonachi_LFSR/Subsystem/16bLFSR1/9 ==
  reg_in : Inport
  Delay : Delay  DelayLength=1  InitialCondition=0  SampleTime=Ts
  reg_out : Outport
  wires:
  Delay/1 -> reg_out/1
  reg_in/1 -> Delay/1
